simulink model "Grid_connected_windfarm_multiple_PMSGs"  (R2019a)
settings: Solver=VariableStepAuto  StartTime=0.0  StopTime=4  RelTol=1e-3  EnableMultiTasking=on
InitFcn:
  | clear all;clc;
  | int5
values from neighbouring files (symbols this model uses):
  Cdc = PMSG(:,16)./w0    [int5.m]
  Id_fault = zeros(N_PMSG,1)    [int5.m]
  Iq_fault = Id_fault    [int5.m]
  Ki_Id = PMSG(:,22)    [int5.m]
  Ki_Iq = PMSG(:,24)    [int5.m]
  Ki_pll = w0.*PMSG(:,26)    [int5.m]
  Ki_Q = PMSG(:,20)    [int5.m]
  Ki_Vdc = PMSG(:,18)    [int5.m]
  Kp_Id = PMSG(:,21)    [int5.m]
  Kp_Iq = PMSG(:,23)    [int5.m]
  Kp_pll = w0.*PMSG(:,25)    [int5.m]
  Kp_Q = PMSG(:,19)    [int5.m]
  Kp_Vdc = PMSG(:,17)    [int5.m]
  Mnet_RL = RL*ones(N_PMSG,N_PMSG)    [int5.m]
  Mnet_XL = Mnet_XL+x    [int5.m]
  Po_ref = zeros(N_PMSG,1)    [int5.m]
  Qo_ref = zeros(N_PMSG,1)    [int5.m]
  Vdc_ref = PMSG(:,14)    [int5.m]
  w0 = 2*3.14*50*ones(N_PMSG,1)    [int5.m]
  Xf = PMSG(:,15)    [int5.m]
libraries: powerlib x1
settings Model: Creator=Gaozhen  LastModifiedBy=15481
settings DataIOCC: InitialState=xFinal  LimitDataPoints=on  SaveOperatingPoint=on  SaveFormat=Array  ReturnWorkspaceOutputs=off
settings OptimizationCC: LifeSpan=inf
settings DebuggingCC: SolverPrmCheckMsg=warning  SFUnexpectedBacktrackingDiag=warning  SFNoUnconditionalDefaultTransitionDiag=warning  SFExecutionAtInitializationDiag=none  ArithmeticOperatorsInVariantConditions=warning
settings HardwareCC: ProdBitPerPointer=32  ProdBitPerSizeT=32  ProdBitPerPtrDiffT=32  ProdLargestAtomicFloat=None  ProdIntDivRoundTo=Undefined  ProdEndianess=Unspecified  ProdWordSize=32  ProdHWDeviceType=32-bit Generic
settings ModelReferenceCC: PropagateSignalLabelsOutOfModel=off
settings SFSimCC: SimUseLocalCustomCode=off
settings RTWCC: RTWUseLocalCustomCode=off
settings CodeAppCC: StateflowObjectComments=on
settings GRTTargetCC: TargetLangStandard=C89/C90 (ANSI)  GeneratePreprocessorConditionals=Disable all
settings ConfigComp: CovMetricSettings=dw  CovHtmlReporting=on  CovSaveCumulativeToWorkspaceVar=on  CovSaveSingleToWorkspaceVar=on  CovExternalEMLEnable=off  CovSFcnEnable=off
settings SimscapeCC: SimscapeNormalizeSystem=off

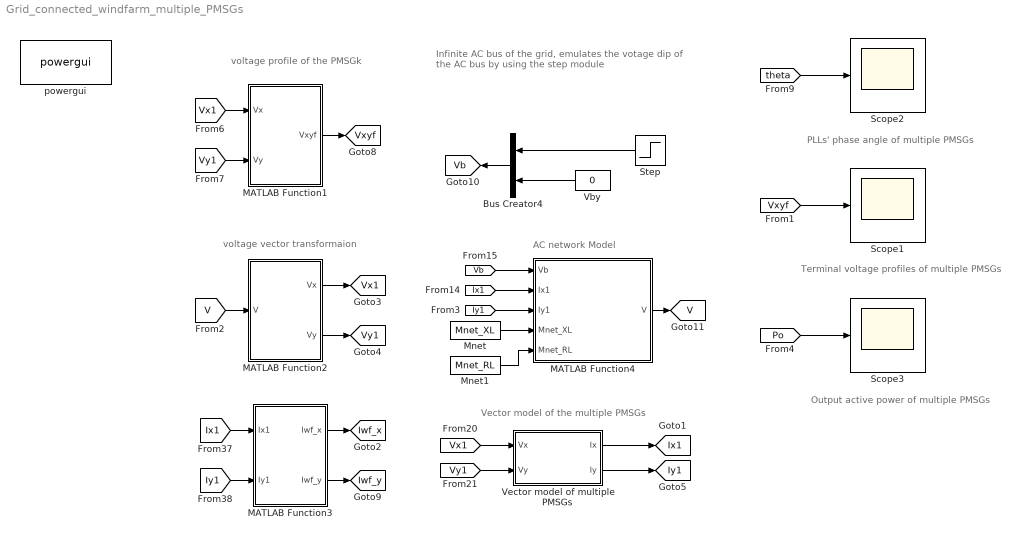
== system Grid_connected_windfarm_multiple_PMSGs ==
  note: Output active power of multiple PMSGs
  note: Vector model of the multiple PMSGs
  note: AC network Model
  note: Infinite AC bus of the grid, emulates the votage dip of the AC bus by using the step module
  note: voltage profile of the PMSGk
  note: voltage vector transformaion
  note: Terminal voltage profiles of multiple PMSGs
  note: PLLs' phase angle of multiple PMSGs
  Bus Creator4 : BusCreator  Inputs=2
  MATLAB Function1 : MATLAB Function  TreatAsAtomicUnit=on
  MATLAB Function2 : MATLAB Function  TreatAsAtomicUnit=on
  MATLAB Function3 : MATLAB Function  TreatAsAtomicUnit=on
  MATLAB Function4 : MATLAB Function  TreatAsAtomicUnit=on
  Mnet : Constant  Value=Mnet_XL
  Mnet1 : Constant  Value=Mnet_RL
  Scope1 : Scope
  Scope2 : Scope
  Scope3 : Scope
  Step : Step  Time=2  Before=1  After=0.35  SampleTime=0
  Vby : Constant  Value=0
  Vector model of multiple PMSGs : Subsystem
      mask Display: image('windfarm_figure.jpg');
  powergui : powerlib/powergui  Priority=1  SimulationMode=Discrete  SampleTime=1e-3  frequency=60  Iterations=50  frequencyindice=60  Pbase=100e6  ErrMax=1e-4  UnitsV=kV  UnitsW=MW  buscounter=0  FunctionMessages=off  echomessages=off  EnableUseOfTLC=off  CurrentSourceSwitches=off  DisableSnubberDevices=off  DisableRonSwitches=off  DisableVfSwitches=off  DisplayEquations=off  AutomaticDiscreteSolvers=off  SolverType=Tustin  Interpol=off  ExternalGateDelay=off  methode=off  Ts=0  x0status=blocks  SPID=off  SwTol=0  HookPort=off  NonlinearTolerance=0  nMaxIteration=15  ContinueOnMaxIteration=off  RestoreLinks=warning  ResistiveCurrentMeasurement=off  Frange=[0:2:500]  Ylog=off  Xlog=on  ShowGrid=off  save=off  variable=ZData  structure=0  ZoomFFT=off  StartTime=0.0  cycles=1  DisplayStyle=1  fundamental=60  FreqAxis=off  MaxFrequency=1000  frequencyindicesteady=1  RmsSteady=1  display=off
      settings: SourceProductName=Simscape Electrical
  tag scope: Iwf_x=global, Iwf_y=global, Ix1=global, Iy1=global, V=global, Vb=global, Vx1=global, Vxyf=global, Vy1=global
  wires:
  Vector model of multiple PMSGs/1(Ix) -> [Ix1]
  [Iy1] -> MATLAB Function4/3(Iy1)
  [Vy1] -> Vector model of multiple PMSGs/2(Vy)
  [Ix1] -> MATLAB Function4/2(Ix1)
  Bus Creator4/1 -> [Vb]
  MATLAB Function2/2(Vy) -> [Vy1]
  [Vx1] -> Vector model of multiple PMSGs/1(Vx)
  Vby/1 -> Bus Creator4/2
  [Vb] -> MATLAB Function4/1(Vb)
  [Vy1] -> MATLAB Function1/2(Vy)
  MATLAB Function2/1(Vx) -> [Vx1]
  Vector model of multiple PMSGs/2(Iy) -> [Iy1]
  [V] -> MATLAB Function2/1(V)
  MATLAB Function3/1(Iwf_x) -> [Iwf_x]
  [Ix1] -> MATLAB Function3/1(Ix1)
  MATLAB Function4/1(V) -> [V]
  [Iy1] -> MATLAB Function3/2(Iy1)
  [Vx1] -> MATLAB Function1/1(Vx)
  MATLAB Function3/2(Iwf_y) -> [Iwf_y]
  MATLAB Function1/1(Vxyf) -> [Vxyf]
  Step/1 -> Bus Creator4/1
  [theta] -> Scope2/1
  [Vxyf] -> Scope1/1
  [Po] -> Scope3/1
  Mnet/1 -> MATLAB Function4/4(Mnet_XL)
  Mnet1/1 -> MATLAB Function4/5(Mnet_RL)

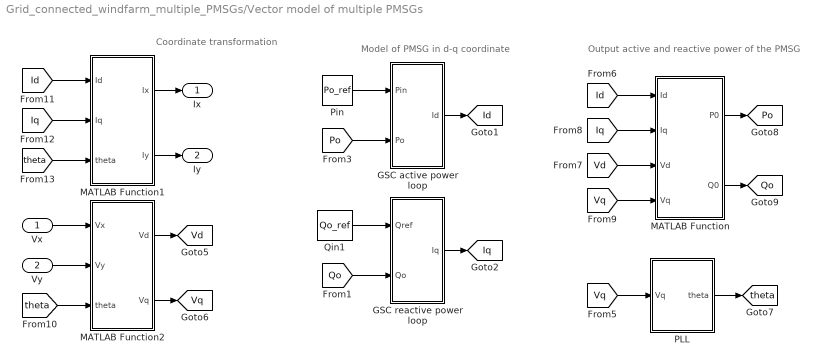
== system Grid_connected_windfarm_multiple_PMSGs/Vector model of multiple PMSGs ==
  note: Output active and reactive power of the PMSG
  note: Model of PMSG in d-q coordinate
  note: Coordinate transformation
  Vx : Inport
  Vy : Inport  Port=2
  "GSC active power loop " : Subsystem
  "GSC reactive power loop " : Subsystem
  MATLAB Function : MATLAB Function  TreatAsAtomicUnit=on
  MATLAB Function1 : MATLAB Function  TreatAsAtomicUnit=on
  MATLAB Function2 : MATLAB Function  TreatAsAtomicUnit=on
  PLL : Subsystem
  Pin : Constant  Value=Po_ref
  Qin1 : Constant  Value=Qo_ref
  Ix : Outport
  Iy : Outport  Port=2
  tag scope: Id=global, Iq=global, Po=global, Qo=global, Vd=global, Vq=global, theta=global
  wires:
  "GSC active power loop "/1(Id) -> [Id]
  [Po] -> "GSC active power loop "/2(Po)
  [Qo] -> "GSC reactive power loop "/2(Qo)
  "GSC reactive power loop "/1(Iq) -> [Iq]
  [Id] -> MATLAB Function1/1(Id)
  [Iq] -> MATLAB Function1/2(Iq)
  [theta] -> MATLAB Function1/3(theta)
  MATLAB Function1/1(Ix) -> Ix/1
  MATLAB Function1/2(Iy) -> Iy/1
  Vx/1 -> MATLAB Function2/1(Vx)
  Vy/1 -> MATLAB Function2/2(Vy)
  [theta] -> MATLAB Function2/3(theta)
  [Vq] -> PLL/1(Vq)
  PLL/1(theta) -> [theta]
  [Id] -> MATLAB Function/1(Id)
  [Iq] -> MATLAB Function/2(Iq)
  [Vd] -> MATLAB Function/3(Vd)
  [Vq] -> MATLAB Function/4(Vq)
  MATLAB Function/2(Q0) -> [Qo]
  MATLAB Function/1(P0) -> [Po]
  MATLAB Function2/1(Vd) -> [Vd]
  MATLAB Function2/2(Vq) -> [Vq]
  Pin/1 -> "GSC active power loop "/1(Pin)
  Qin1/1 -> "GSC reactive power loop "/1(Qref)

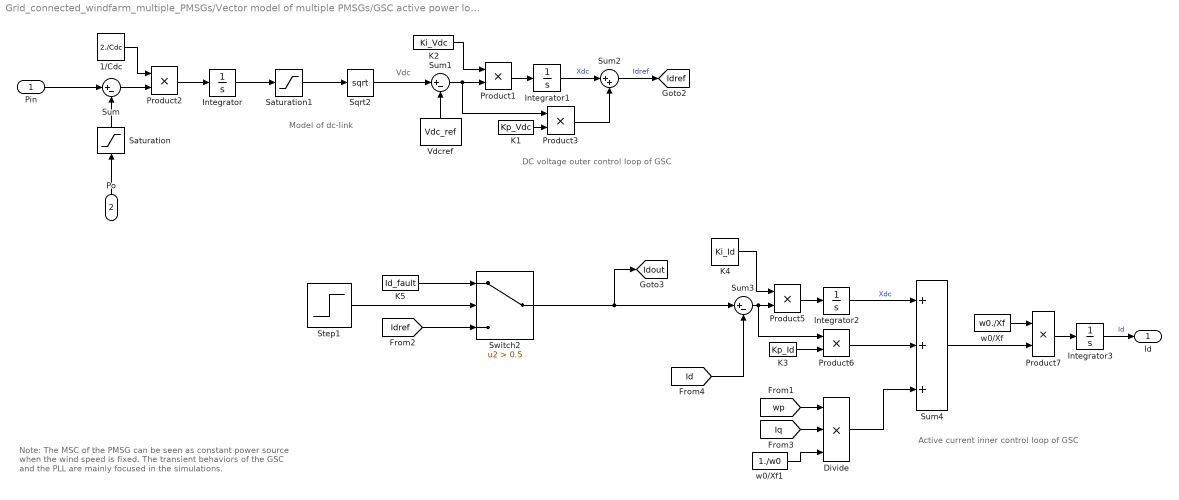
== system Grid_connected_windfarm_multiple_PMSGs/Vector model of multiple PMSGs/GSC active power loop  ==
  note: Active current inner control loop of GSC
  note: DC voltage outer control loop of GSC
  note: Model of dc-link
  note: Note:
      | The MSC of the PMSG can be seen as constant power source
      | when the wind speed is fixed. The transient behaviors of the
      | GSC and the PLL are mainly focused in the simulations.
  note: Vdc
  Pin : Inport
  Po : Inport  Port=2
  1/Cdc : Constant  Value=2./Cdc
  Divide : Product  Inputs=***
  Integrator : Integrator  InitialCondition=1
  Integrator1 : Integrator  InitialCondition=0.02
  Integrator2 : Integrator
  Integrator3 : Integrator  InitialCondition=0.02
  K1 : Constant  Value=Kp_Vdc
  K2 : Constant  Value=Ki_Vdc
  K3 : Constant  Value=Kp_Id
  K4 : Constant  Value=Ki_Id
  K5 : Constant  Value=Id_fault
  Product{1..3,5..7} (6 alike) : Product
  Saturation : Saturate  UpperLimit=1  LowerLimit=-1
  Saturation1 : Saturate  UpperLimit=5  LowerLimit=0
  Sqrt2 : Sqrt  SaturateOnIntegerOverflow=on
  Step1 : Step  Time=2  SampleTime=0
  Sum : Sum  Inputs=|+-
  Sum1 : Sum  Inputs=|+-
  Sum2 : Sum  Inputs=|++
  Sum3 : Sum  Inputs=|+-
  Sum4 : Sum  Inputs=+++
  Switch2 : Switch  Criteria=u2 > Threshold  Threshold=0.5
  Vdcref : Constant  Value=Vdc_ref
  w0/Xf : Constant  Value=w0./Xf
  w0/Xf1 : Constant  Value=1./w0
  Id : Outport
  tag scope: Idout=global, Idref=global
  wires:
  Product2/1 -> Integrator/1
  Pin/1 -> Sum/1
  Product3/1 -> Sum2/2
  Integrator1/1 -> Sum2/1  "Xdc"
  K1/1 -> Product3/2
  Product1/1 -> Integrator1/1
  Sum1/1 -> Product1/2, Product3/1
  K2/1 -> Product1/1
  Sum/1 -> Product2/2
  Vdcref/1 -> Sum1/2
  1/Cdc/1 -> Product2/1
  Product5/1 -> Integrator2/1
  K3/1 -> Product6/2
  K4/1 -> Product5/1
  Sum3/1 -> Product6/1, Product5/2
  Integrator2/1 -> Sum4/1  "Xdc"
  Product6/1 -> Sum4/2
  Product7/1 -> Integrator3/1
  Sum4/1 -> Product7/2
  w0/Xf/1 -> Product7/1
  Integrator3/1 -> Id/1  "Id"
  Saturation/1 -> Sum/2
  Sqrt2/1 -> Sum1/1
  Po/1 -> Saturation/1
  Integrator/1 -> Saturation1/1
  Saturation1/1 -> Sqrt2/1
  Sum2/1 -> [Idref]  "Idref"
  [wp] -> Divide/1
  [Iq] -> Divide/2
  w0/Xf1/1 -> Divide/3
  Divide/1 -> Sum4/3
  [Id] -> Sum3/2
  Step1/1 -> Switch2/2
  [Idref] -> Switch2/3
  Switch2/1 -> [Idout], Sum3/1
  K5/1 -> Switch2/1

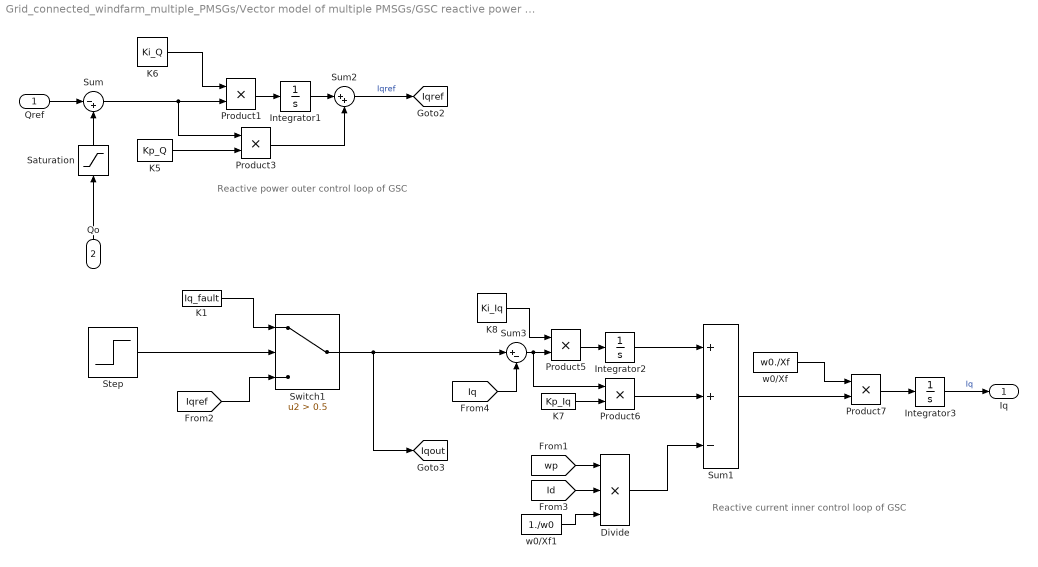
== system Grid_connected_windfarm_multiple_PMSGs/Vector model of multiple PMSGs/GSC reactive power loop  ==
  note: Reactive current inner control loop of GSC
  note: Reactive power outer control loop of GSC
  Qref : Inport
  Qo : Inport  Port=2
  Divide : Product  Inputs=***
  Integrator1 : Integrator  InitialCondition=-0.005
  Integrator2 : Integrator
  Integrator3 : Integrator  InitialCondition=-0.005
  K1 : Constant  Value=Iq_fault
  K5 : Constant  Value=Kp_Q
  K6 : Constant  Value=Ki_Q
  K7 : Constant  Value=Kp_Iq
  K8 : Constant  Value=Ki_Iq
  Product{1,3,5..7} (5 alike) : Product
  Saturation : Saturate  UpperLimit=10  LowerLimit=-10
  Step : Step  Time=2  SampleTime=0
  Sum : Sum  Inputs=|-+
  Sum1 : Sum  Inputs=++-
  Sum2 : Sum  Inputs=|++
  Sum3 : Sum  Inputs=|+-
  Switch1 : Switch  Criteria=u2 > Threshold  Threshold=0.5
  w0/Xf : Constant  Value=w0./Xf
  w0/Xf1 : Constant  Value=1./w0
  Iq : Outport
  tag scope: Iqout=global, Iqref=global
  wires:
  Integrator3/1 -> Iq/1  "Iq"
  w0/Xf/1 -> Product7/1
  Product7/1 -> Integrator3/1
  Sum3/1 -> Product5/2, Product6/1
  K8/1 -> Product5/1
  K7/1 -> Product6/2
  Product5/1 -> Integrator2/1
  K6/1 -> Product1/1
  Sum/1 -> Product1/2, Product3/1
  Product1/1 -> Integrator1/1
  K5/1 -> Product3/2
  Integrator1/1 -> Sum2/1
  Product3/1 -> Sum2/2
  Saturation/1 -> Sum/2
  Qref/1 -> Sum/1
  Qo/1 -> Saturation/1
  Step/1 -> Switch1/2
  [Iqref] -> Switch1/3
  Switch1/1 -> [Iqout], Sum3/1
  Sum2/1 -> [Iqref]  "Iqref"
  Divide/1 -> Sum1/3
  w0/Xf1/1 -> Divide/3
  [wp] -> Divide/1
  [Id] -> Divide/2
  Integrator2/1 -> Sum1/1
  Product6/1 -> Sum1/2
  Sum1/1 -> Product7/2
  [Iq] -> Sum3/2
  K1/1 -> Switch1/1

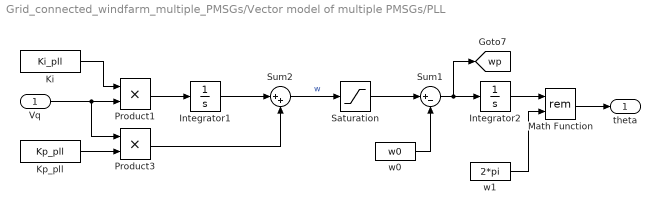
== system Grid_connected_windfarm_multiple_PMSGs/Vector model of multiple PMSGs/PLL ==
  Vq : Inport
  Integrator1 : Integrator  InitialCondition=2*pi*50
  Integrator2 : Integrator  InitialCondition=0.9
  Ki : Constant  Value=Ki_pll
  Kp_pll : Constant  Value=Kp_pll
  Math Function : Math  Operator=rem  SaturateOnIntegerOverflow=on
  Product1 : Product
  Product3 : Product
  Saturation : Saturate  UpperLimit=w0*1.2  LowerLimit=w0*0.8
  Sum1 : Sum  Inputs=|+-
  Sum2 : Sum  Inputs=|++
  w0 : Constant  Value=w0
  w1 : Constant  Value=2*pi
  theta : Outport
  tag scope: wp=global
  wires:
  Product3/1 -> Sum2/2
  Product1/1 -> Integrator1/1
  Ki/1 -> Product1/1
  w0/1 -> Sum1/2
  Sum1/1 -> [wp], Integrator2/1
  Vq/1 -> Product1/2, Product3/1
  Kp_pll/1 -> Product3/2
  Integrator1/1 -> Sum2/1
  Integrator2/1 -> Math Function/1
  w1/1 -> Math Function/2
  Math Function/1 -> theta/1
  Sum2/1 -> Saturation/1  "w"
  Saturation/1 -> Sum1/1

== matlab function Grid_connected_windfarm_multiple_PMSGs/Vector model of multiple PMSGs/MATLAB Function ==
  data: Id input; Iq input; P0 output; Vd input; Vq input; Q0 output
function [P0,Q0] = power(Id,Iq,Vd,Vq)
%% PMSG输出有功
P0=Id.*Vd+Iq.*Vq;
%% PMSG输出无功
Q0=Id.*Vq-Iq.*Vd;

== matlab function Grid_connected_windfarm_multiple_PMSGs/Vector model of multiple PMSGs/MATLAB Function1 ==
  data: Id input; Iq input; Ix output; theta input; Iy output
function [Ix,Iy] = Rdq_xy(Id,Iq,theta)
%% 
Ix=Id.*cos(theta)-Iq.*sin(theta);
Iy=Id.*sin(theta)+Iq.*cos(theta);

== matlab function Grid_connected_windfarm_multiple_PMSGs/Vector model of multiple PMSGs/MATLAB Function2 ==
  data: Vx input; Vy input; Vd output; theta input; Vq output
function [Vd,Vq] = Rxy_dc(Vx,Vy,theta)
%% 
Vd=Vx.*cos(theta)+Vy.*sin(theta);
Vq=-Vx.*sin(theta)+Vy.*cos(theta);

== matlab function Grid_connected_windfarm_multiple_PMSGs/MATLAB Function1 ==
  data: Vx input; Vy input; Vxyf output
function Vxyf = mag_V(Vx,Vy)
Vxyf=sqrt(Vx.^2+Vy.^2);% calculate the amplitude of the terminal voltage of kth PMSG

== matlab function Grid_connected_windfarm_multiple_PMSGs/MATLAB Function2 ==
  data: V input; Vx output; Vy output
function [Vx,Vy] = voltage(V)
N=0.5*length(V);% N represnets the number of the PMSGs in the wind farm
%% Vx Vy initialization
Vx=zeros(N,1);
Vy=zeros(N,1);
%% Generate Vx vector and Vy vector from the voltage vector V；
% V=[Vx1;Vy1;Vx2;Vy2 ... VxN;VyN];
% Vx=[Vx1;Vx2 ... VxN];Vy=[Vy1;Vy2 ... VyN];
for k=1:N
    Vx(k)=V(2*k-1);
    Vy(k)=V(2*k);
end

== matlab function Grid_connected_windfarm_multiple_PMSGs/MATLAB Function4 ==
  data: Vb input; Ix1 input; Iy1 input; V output; Mnet_XL input; Mnet_RL input
function V = WF_Net(Vb,Ix1,Iy1,Mnet_XL,Mnet_RL)
I1=[Ix1;Iy1];
%% Initialization
H1=[0 -1;1 0];H2=[1 0;0 1];% 
M=kron(Mnet_XL,H1)+kron(Mnet_RL,H2);% M is 2N*2N network matrix
%% terminal voltage and current relationship of PMSG；Vb=[Vbx;0] is the voltage bus of the AC grid.
N=length(Ix1);% N is the number of the PMSGs in wind farm
Vb_2N=zeros(2*N,1);% Initialization
I=zeros(2*N,1);
%% Vb_2N=[Vb Vb ... Vb]is the 2N dimensional vector；
for k=1:N
    Vb_2N(2*k-1)=Vb(1);
    Vb_2N(2*k)=Vb(2);
end
for k=1:N
    I(2*k-1)=I1(k);
    I(2*k)=I1(k+N);
end
V = M*I+Vb_2N;

== matlab function Grid_connected_windfarm_multiple_PMSGs/MATLAB Function3 ==
  data: Ix1 input; Iy1 input; Iwf_x output; Iwf_y output
function [Iwf_x,Iwf_y] = mag_V(Ix1,Iy1)
N=0.5*length(Ix1);% 风机台数N
%% Ix Vy初始化
Iwf_x=0;
Iwf_y=0;
for k=1:N
    Iwf_x=Iwf_x+Ix1(k);
    Iwf_y=Iwf_y+Iy1(k);
end
